simulink library "boatGroundStation_cl"  (R2020a)
settings: Solver=VariableStepAuto  StartTime=0.0  StopTime=10.0  RelTol=1e-3
undefined symbols (not defined in the file): gndStn, initGndStnPos, tow_speed, x_init
libraries: eulAng2RotMat_ul x1, firstOrdTrnsThm_ul x1
settings Model: Creator=M.Cobb  LastModifiedBy=adabney
settings DataIOCC: ReturnWorkspaceOutputs=off
settings DebuggingCC: ArithmeticOperatorsInVariantConditions=warning
settings SFSimCC: CustomCodeUndefinedFunction=UseInterfaceOnly

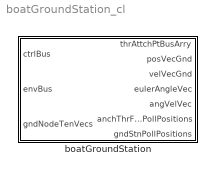
== system boatGroundStation_cl ==
  boatGroundStation : Subsystem  VariantControl=VSS_groundStation_raftGroundStation  mask{gs=gndStn}
      mask prompts: gs "Ground station object"

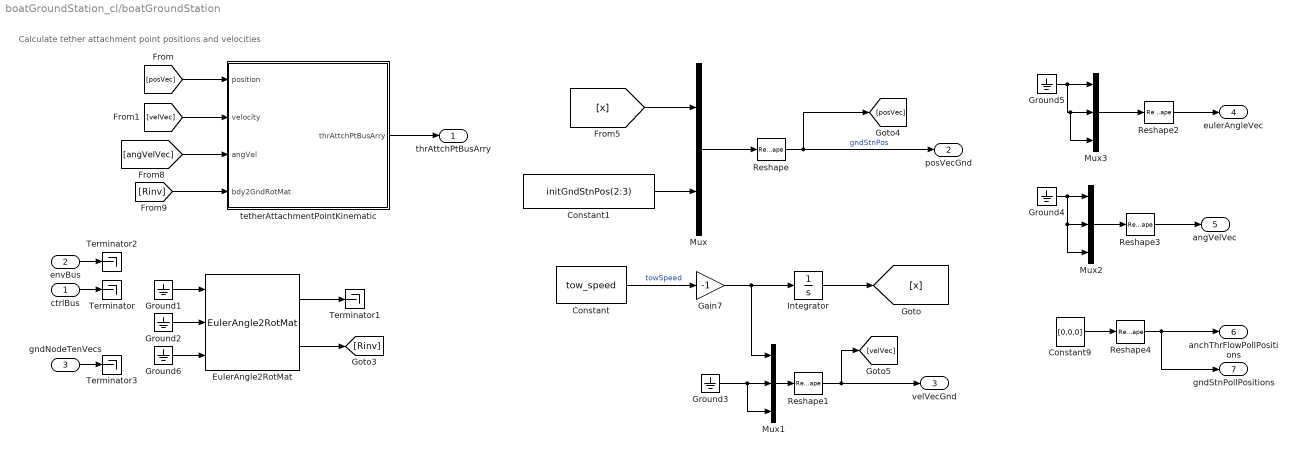
== system boatGroundStation_cl/boatGroundStation ==
  note: Calculate tether attachment point positions and velocities
  ctrlBus : Inport  OutDataTypeStr=Bus: gndStnCtrlBus
  envBus : Inport  Port=2  OutDataTypeStr=Bus: envBus
  gndNodeTenVecs : Inport  Port=3
  Constant : Constant  Value=tow_speed
  Constant1 : Constant  Value=initGndStnPos(2:3)
  Constant9 : Constant  Value=[0,0,0]
  EulerAngle2RotMat : eulAng2RotMat_ul/EulerAngle2RotMat  SystemSampleTime=-1  Latency=0  AutoFrameSizeCalculation=off
  Gain7 : Gain  Gain=-1
  Ground{1..6} (6 alike) : Ground
  Integrator : Integrator  InitialCondition=x_init
  Mux : Mux  Inputs=2
  Mux1 : Mux  Inputs=3
  Mux2 : Mux  Inputs=3
  Mux3 : Mux  Inputs=3
  Reshape{,1..4} (5 alike) : Reshape  OutputDimensionality=Column vector (2-D)
  Terminator{,1..3} (4 alike) : Terminator
  tetherAttachmentPointKinematic : Subsystem  InitFcn=thrAttachPtKinematics_init  mask{atchPts=[0 0 0]}
      mask prompts: atchPts "Tether attachment point vec in platform frame"
      mask init:
      | thrAttachPtKinematics_init
  thrAttchPtBusArry : Outport  VectorParamsAs1DForOutWhenUnconnected=off
  posVecGnd : Outport  Port=2  VectorParamsAs1DForOutWhenUnconnected=off
  velVecGnd : Outport  Port=3  VectorParamsAs1DForOutWhenUnconnected=off
  eulerAngleVec : Outport  Port=4  VectorParamsAs1DForOutWhenUnconnected=off
  angVelVec : Outport  Port=5  VectorParamsAs1DForOutWhenUnconnected=off
  anchThrFlowPollPositions : Outport  Port=6  VectorParamsAs1DForOutWhenUnconnected=off
  gndStnPollPositions : Outport  Port=7  VectorParamsAs1DForOutWhenUnconnected=off
  wires:
  tetherAttachmentPointKinematic/1(thrAttchPtBusArry) -> thrAttchPtBusArry/1
  [posVec] -> tetherAttachmentPointKinematic/1(position)
  [velVec] -> tetherAttachmentPointKinematic/2(velocity)
  Reshape/1 -> [posVec], posVecGnd/1  "gndStnPos"
  Reshape1/1 -> velVecGnd/1, [velVec]
  Reshape2/1 -> eulerAngleVec/1
  Reshape3/1 -> angVelVec/1
  Integrator/1 -> [x]
  Constant/1 -> Gain7/1  "towSpeed"
  [x] -> Mux/1
  Mux/1 -> Reshape/1
  EulerAngle2RotMat/2 -> [Rinv]
  EulerAngle2RotMat/1 -> Terminator1/1
  Ground6/1 -> EulerAngle2RotMat/3
  Ground1/1 -> EulerAngle2RotMat/1
  Ground2/1 -> EulerAngle2RotMat/2
  ctrlBus/1 -> Terminator/1
  envBus/1 -> Terminator2/1
  gndNodeTenVecs/1 -> Terminator3/1
  Mux1/1 -> Reshape1/1
  Mux2/1 -> Reshape3/1
  Ground4/1 -> Mux2/3, Mux2/2, Mux2/1
  Mux3/1 -> Reshape2/1
  Ground5/1 -> Mux3/3, Mux3/2, Mux3/1
  Constant1/1 -> Mux/2
  [angVelVec] -> tetherAttachmentPointKinematic/3(angVel)
  [Rinv] -> tetherAttachmentPointKinematic/4(bdy2GndRotMat)
  Reshape4/1 -> anchThrFlowPollPositions/1, gndStnPollPositions/1
  Constant9/1 -> Reshape4/1
  Gain7/1 -> Mux1/1, Integrator/1
  Ground3/1 -> Mux1/3, Mux1/2

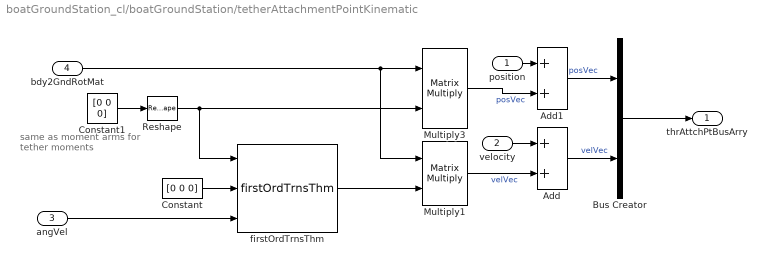
== system boatGroundStation_cl/boatGroundStation/tetherAttachmentPointKinematic ==
  note: same as moment arms
      | for tether moments
  position : Inport
  velocity : Inport  Port=2
  angVel : Inport  Port=3
  bdy2GndRotMat : Inport  Port=4
  Add : Sum
  Add1 : Sum
  Bus Creator : BusCreator  Inputs=2  OutDataTypeStr=Bus: thrAttachPtKinematicsBus  NonVirtualBus=on
  Constant : Constant  Value=[0 0 0]
  Constant1 : Constant  Value=[0 0 0]
  Multiply1 : Product  Multiplication=Matrix(*)
  Multiply3 : Product  Multiplication=Matrix(*)
  Reshape : Reshape  OutputDimensionality=Column vector (2-D)
  firstOrdTrnsThm : firstOrdTrnsThm_ul/firstOrdTrnsThm  SystemSampleTime=-1  Latency=0  AutoFrameSizeCalculation=off
  thrAttchPtBusArry : Outport  VectorParamsAs1DForOutWhenUnconnected=off
  wires:
  Reshape/1 -> firstOrdTrnsThm/1, Multiply3/2
  Multiply3/1 -> Add1/2  "posVec"
  Multiply1/1 -> Add/2  "velVec"
  velocity/1 -> Add/1
  position/1 -> Add1/1
  Bus Creator/1 -> thrAttchPtBusArry/1
  Constant1/1 -> Reshape/1
  angVel/1 -> firstOrdTrnsThm/3
  firstOrdTrnsThm/1 -> Multiply1/2
  Constant/1 -> firstOrdTrnsThm/2
  bdy2GndRotMat/1 -> Multiply3/1, Multiply1/1
  Add/1 -> Bus Creator/2  "velVec"
  Add1/1 -> Bus Creator/1  "posVec"
